simulink library "camera_update_lib"  (R2016b)
settings: Solver=ode45  StartTime=0.0  StopTime=10.0  RelTol=1e-3  EnableMultiTasking=on
undefined symbols (not defined in the file): accel_bias, ase_aug_state_bitmask, ase_hr_distance_r, ase_hr_r_mag, ase_local_mode_docking, ase_local_mode_map, ase_local_mode_perching, ase_minumum_resid_thresh, ase_ml_num_features, ase_of_num_aug, ase_of_num_features, ase_status_converged, ase_total_num_states, gyro_bias, hr_P_hr_ISS_ISS, hr_quat_ISS2hr, kfl_status, ml_mahal_distance, ml_P_cam_ISS_ISS, ml_quat_ISS2cam, of_mahal_distance, of_P_cam_ISS_ISS, of_quat_ISS2cam, P_EST_ISS_ISS, quat_ISS2B, tun_abp_q_body2dockcam, tun_abp_q_body2navcam, tun_abp_q_body2perchcam, tun_ase_dock_r_mag, tun_ase_dockcam_distortion, tun_ase_dockcam_inv_focal_length, tun_ase_enable_of, tun_ase_mahal_distance_max, tun_ase_map_error, tun_ase_min_hr_meas, tun_ase_min_ml_meas, tun_ase_min_of_meas, tun_ase_ml_forward_projection_time, tun_ase_navcam_distortion, tun_ase_navcam_inv_focal_length, tun_ase_of_r_mag, tun_ase_vis_r_mag, tun_ase_vocam_inv_focal_length, update_ML_features_cnt, update_OF_tracks_cnt, V_B_ISS_ISS
libraries: simulink x13, camera_update_lib x1
(part 2 of 2)

== matlab function camera_update_lib/camera_update/Absolute_Update/ML Update/Compute Residual and H matrix/ML_Compute_Residual_and_H/Compute Residual and H ==
  data: r_out output size=[6 1]; error_out output; H_out output size=[6 ase_total_num_states]; R_mat output size=[6 6]; numFeatures output; inv_focal_length input; distortion input; mahal_dists output size=[ase_ml_num_features 1]; ml_P_cam_ISS_ISS input; ml_quat_ISS2cam input; is_converged input; omega input; velocity input; L input; O input; valid input; P_in input; tun_ase_mahal_distance_max parameter; tun_ase_min_ml_meas parameter; ase_of_num_aug parameter; ase_ml_num_features parameter; tun_ase_vis_r_mag parameter; tun_ase_map_error parameter; q_body2cam input; tun_ase_ml_forward_projection_time parameter; ML_update input; tun_ase_dock_r_mag parameter
function [r_out, error_out, H_out, R_mat, numFeatures, mahal_dists] = compute_ml_residual_and_h(inv_focal_length, distortion, ml_P_cam_ISS_ISS, ml_quat_ISS2cam, is_converged, omega, velocity, L, O, valid, P_in, tun_ase_mahal_distance_max, tun_ase_min_ml_meas, ase_of_num_aug, ase_ml_num_features, tun_ase_vis_r_mag, tun_ase_map_error, q_body2cam, tun_ase_ml_forward_projection_time, ML_update, tun_ase_dock_r_mag)
%#codegen
[r_out, error_out, H_out, R_mat, numFeatures, mahal_dists] = eml_compute_ml_residual_and_h(inv_focal_length, distortion, ml_P_cam_ISS_ISS, ml_quat_ISS2cam, is_converged, omega, velocity, L, O, valid, P_in, tun_ase_mahal_distance_max, tun_ase_min_ml_meas, ase_of_num_aug, ase_ml_num_features, tun_ase_vis_r_mag, tun_ase_map_error, q_body2cam', tun_ase_ml_forward_projection_time, ML_update, tun_ase_dock_r_mag);
